simulink model "AMR_LidarLoc_UDP_decoder_24a"  (R2024a)
settings: configuration reference "SharedConfig" (kept outside this file)
undefined symbols (not defined in the file): tstep
libraries: slrealtimeutilitieslib x6
settings Model: DataDictionary=configuration_dictionary.sldd  Creator=anderson.bordin  LastModifiedBy=matlab.cut
settings ConfigSetRef: SourceName=SharedConfig

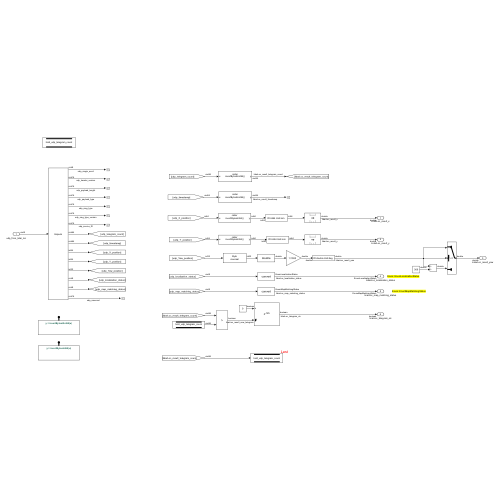
[thumbnail: Simulink's stored preview of the top-level diagram]
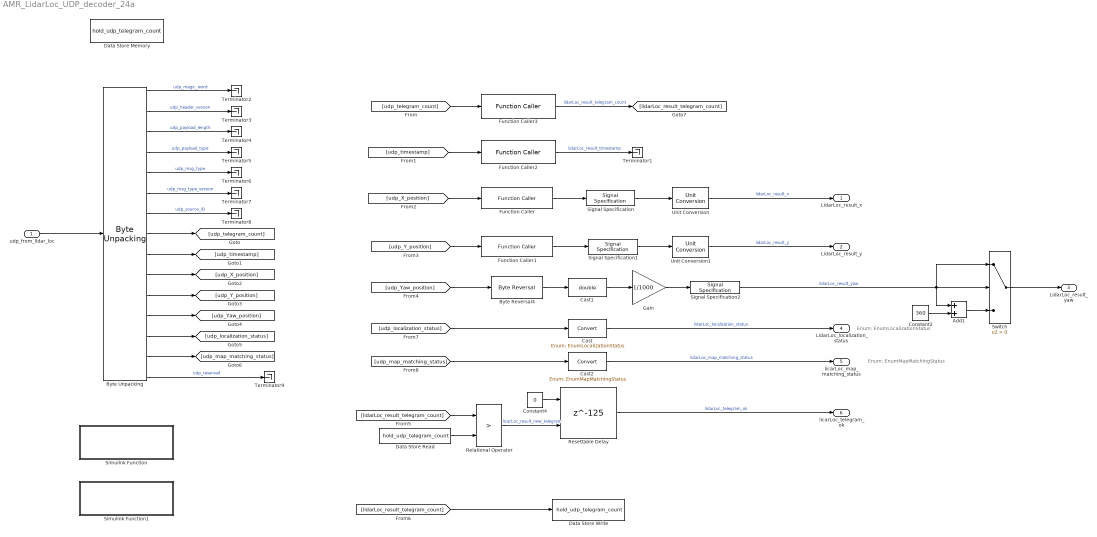
== system AMR_LidarLoc_UDP_decoder_24a ==
  note: Enum: EnumLocalizationStatus
  note: Enum: EnumMapMatchingStatus
  udp_from_lidar_loc : Inport  OutDataTypeStr=uint8  PortDimensions=56
  Add1 : Sum
  Byte Reversal4 : slrealtimeutilitieslib/Byte Reversal  numInp=1
  Byte Unpacking : slrealtimeutilitieslib/Byte Unpacking  MaskUnpackedDataTypes={['uint8'],'uint16','uint16','uint16','uint16','uint16','uint16','uint64','uint64','int64','int64','int32','uint8','uint8','uint16'}  MaskUnpackedDataSizes={[4],1,1,1,1,1,1,1,1,1,1,1,1,1,1}  MaskAlignment=1
  Cast : DataTypeConversion  OutDataTypeStr=Enum: EnumLocalizationStatus  SaturateOnIntegerOverflow=off  RndMeth=Floor
  Cast1 : DataTypeConversion  OutDataTypeStr=double  SaturateOnIntegerOverflow=off  RndMeth=Floor
  Cast2 : DataTypeConversion  OutDataTypeStr=Enum: EnumMapMatchingStatus  SaturateOnIntegerOverflow=off  RndMeth=Floor
  Constant2 : Constant  Value=360
  Constant4 : Constant  Value=0  OutDataTypeStr=boolean
  Data Store Memory : DataStoreMemory  DataStoreName=hold_udp_telegram_count  WriteAfterWriteMsg=warning  ShowAdditionalParam=off  OutDataTypeStr=uint64  Dimensions=1
      settings: LockScale=on
  Data Store Read : DataStoreRead  DataStoreName=hold_udp_telegram_count  DataStoreElements=hold_udp_telegram_count  IndexOptions=Index vector (dialog)  Indices=1  OutputSizes=1
  Data Store Write : DataStoreWrite  ExecutionOrder=Last  DataStoreName=hold_udp_telegram_count  DataStoreElements=hold_udp_telegram_count  IndexOptions=Index vector (dialog)  Indices=1  OutputSizes=1
  Function Caller : FunctionCaller  FunctionPrototype=y = invertBytesInt64(u)  InputArgumentSpecifications=<Enter example>  OutputArgumentSpecifications=<Enter example>
  Function Caller1 : FunctionCaller  FunctionPrototype=y = invertBytesInt64(u)  InputArgumentSpecifications=<Enter example>  OutputArgumentSpecifications=<Enter example>
  Function Caller2 : FunctionCaller  FunctionPrototype=y = invertBytesUint64(u)  InputArgumentSpecifications=<Enter example>  OutputArgumentSpecifications=<Enter example>
  Function Caller3 : FunctionCaller  FunctionPrototype=y = invertBytesUint64(u)  InputArgumentSpecifications=<Enter example>  OutputArgumentSpecifications=<Enter example>
  Gain : Gain  Gain=1/1000  OutDataTypeStr=double
  Relational Operator : RelationalOperator  Operator=>  OutDataTypeStr=boolean  RndMeth=Simplest  InputSameDT=off
  Resettable Delay : Delay  DelayLength=125  InitialCondition=1  ExternalReset=Rising  SampleTime=tstep
      settings: InputPortMap=u0,r5
  Signal Specification : SignalSpecification  OutDataTypeStr=int64  Unit=mm
  Signal Specification1 : SignalSpecification  OutDataTypeStr=int64  Unit=mm
  Signal Specification2 : SignalSpecification  OutDataTypeStr=double  Unit=deg
  Simulink Function : Subsystem  TreatAsAtomicUnit=on
  Simulink Function1 : Subsystem  TreatAsAtomicUnit=on
  Switch : Switch  Criteria=u2 > Threshold  SaturateOnIntegerOverflow=off  InputSameDT=off
  Terminator{1..9} (9 alike) : Terminator
  Unit Conversion : UnitConversion  OutputType=Inherit: Inherit via back propagation
  Unit Conversion1 : UnitConversion  OutputType=Inherit: Inherit via back propagation
  LidarLoc_result_x : Outport  OutDataTypeStr=double  Unit=m
  LidarLoc_result_y : Outport  Port=2  OutDataTypeStr=double  Unit=m
  LidarLoc_result_yaw : Outport  Port=3  OutDataTypeStr=double  Unit=deg
  LidarLoc_localization_status : Outport  Port=4  OutDataTypeStr=Enum: EnumLocalizationStatus
  licarLoc_map_matching_status : Outport  Port=5  OutDataTypeStr=Enum: EnumMapMatchingStatus
  licarLoc_telegram_ok : Outport  Port=6  OutDataTypeStr=boolean
  wires:
  udp_from_lidar_loc/1 -> Byte Unpacking/1
  Function Caller3/1 -> [lidarLoc_result_telegram_count]  "lidarLoc_result_telegram_count"
  Function Caller2/1 -> Terminator1/1  "lidarLoc_result_timestamp"
  Function Caller/1 -> Signal Specification/1
  Byte Reversal4/1 -> Cast1/1
  Byte Unpacking/1 -> Terminator2/1  "udp_magic_word"
  Byte Unpacking/2 -> Terminator3/1  "udp_header_version"
  Byte Unpacking/3 -> Terminator4/1  "udp_payload_length"
  Byte Unpacking/4 -> Terminator5/1  "udp_payload_type"
  Byte Unpacking/5 -> Terminator6/1  "udp_msg_type"
  Byte Unpacking/6 -> Terminator7/1  "udp_msg_type_version"
  Byte Unpacking/7 -> Terminator8/1  "udp_source_ID"
  Byte Unpacking/15 -> Terminator9/1  "udp_reserved"
  Byte Unpacking/8 -> [udp_telegram_count]
  Byte Unpacking/9 -> [udp_timestamp]
  Byte Unpacking/10 -> [udp_X_position]
  Byte Unpacking/11 -> [udp_Y_position]
  Byte Unpacking/12 -> [udp_Yaw_position]
  Byte Unpacking/14 -> [udp_map_matching_status]
  Byte Unpacking/13 -> [udp_localization_status]
  [udp_telegram_count] -> Function Caller3/1
  [udp_X_position] -> Function Caller/1
  [udp_timestamp] -> Function Caller2/1
  [udp_Y_position] -> Function Caller1/1
  [udp_Yaw_position] -> Byte Reversal4/1
  Data Store Read/1 -> Relational Operator/2
  Constant4/1 -> Resettable Delay/1
  Relational Operator/1 -> Resettable Delay/2  "licarLoc_result_new_telegram"
  [lidarLoc_result_telegram_count] -> Relational Operator/1
  [lidarLoc_result_telegram_count] -> Data Store Write/1
  [udp_localization_status] -> Cast/1
  [udp_map_matching_status] -> Cast2/1
  Resettable Delay/1 -> licarLoc_telegram_ok/1  "lidarLoc_telegram_ok"
  Cast/1 -> LidarLoc_localization_status/1  "lidarLoc_localization_status"
  Cast2/1 -> licarLoc_map_matching_status/1  "lidarLoc_map_matching_status"
  Signal Specification/1 -> Unit Conversion/1
  Unit Conversion/1 -> LidarLoc_result_x/1  "lidarLoc_result_x"
  Signal Specification1/1 -> Unit Conversion1/1
  Function Caller1/1 -> Signal Specification1/1
  Unit Conversion1/1 -> LidarLoc_result_y/1  "lidarLoc_result_y"
  Signal Specification2/1 -> Add1/1, Switch/1, Switch/2  "lidarLoc_result_yaw"
  Cast1/1 -> Gain/1
  Gain/1 -> Signal Specification2/1
  Add1/1 -> Switch/3
  Constant2/1 -> Add1/2
  Switch/1 -> LidarLoc_result_yaw/1

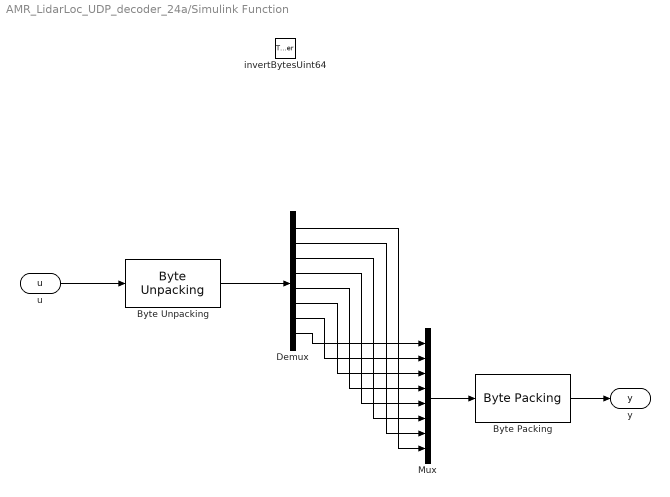
== system AMR_LidarLoc_UDP_decoder_24a/Simulink Function ==
  invertBytesUint64 : TriggerPort  TriggerType=function-call  IsSimulinkFunction=on  FunctionName=invertBytesUint64  FunctionVisibility=scoped  VariantControl=(inherit)
  Byte Packing : slrealtimeutilitieslib/Byte Packing  MaskPackedDataType=uint64  MaskUnpackedDataTypes={['uint8']}  MaskAlignment=1
  Byte Unpacking : slrealtimeutilitieslib/Byte Unpacking  MaskUnpackedDataTypes={['uint8']}  MaskUnpackedDataSizes={[8]}  MaskAlignment=1
  Demux : Demux  Outputs=8
  Mux : Mux  Inputs=8
  u : ArgIn  DisableCoverage=on  OutDataTypeStr=uint64  ArgumentName=u
  y : ArgOut  DisableCoverage=on  OutDataTypeStr=uint64  ArgumentName=y
  wires:
  Demux/5 -> Mux/4
  Demux/4 -> Mux/5
  Demux/8 -> Mux/1
  Byte Unpacking/1 -> Demux/1
  Demux/3 -> Mux/6
  Demux/1 -> Mux/8
  Demux/2 -> Mux/7
  Demux/6 -> Mux/3
  Demux/7 -> Mux/2
  Mux/1 -> Byte Packing/1
  u/1 -> Byte Unpacking/1
  Byte Packing/1 -> y/1

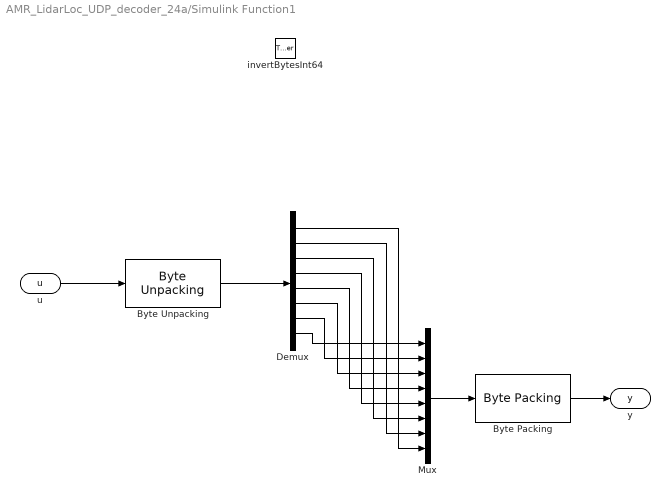
== system AMR_LidarLoc_UDP_decoder_24a/Simulink Function1 ==
  invertBytesInt64 : TriggerPort  TriggerType=function-call  IsSimulinkFunction=on  FunctionName=invertBytesInt64  FunctionVisibility=scoped  VariantControl=(inherit)
  Byte Packing : slrealtimeutilitieslib/Byte Packing  MaskPackedDataType=int64  MaskUnpackedDataTypes={['uint8']}  MaskAlignment=1
  Byte Unpacking : slrealtimeutilitieslib/Byte Unpacking  MaskUnpackedDataTypes={['uint8']}  MaskUnpackedDataSizes={[8]}  MaskAlignment=1
  Demux : Demux  Outputs=8
  Mux : Mux  Inputs=8
  u : ArgIn  DisableCoverage=on  OutDataTypeStr=int64  ArgumentName=u
  y : ArgOut  DisableCoverage=on  OutDataTypeStr=int64  ArgumentName=y
  wires:
  Demux/5 -> Mux/4
  Demux/4 -> Mux/5
  Demux/8 -> Mux/1
  Byte Unpacking/1 -> Demux/1
  Demux/3 -> Mux/6
  Demux/1 -> Mux/8
  Demux/2 -> Mux/7
  Demux/6 -> Mux/3
  Demux/7 -> Mux/2
  u/1 -> Byte Unpacking/1
  Byte Packing/1 -> y/1
  Mux/1 -> Byte Packing/1
